simulink model "projection_test_4D"  (R2018b)
settings: Solver=VariableStepAuto  StartTime=0.0  StopTime=10.0  RelTol=1e-3
undefined symbols (not defined in the file): fswParams
libraries: simulink_extras x6, vrlib x2, L_inf_allocation_lib x1
settings Model: Creator=Taylor  LastModifiedBy=Taylor

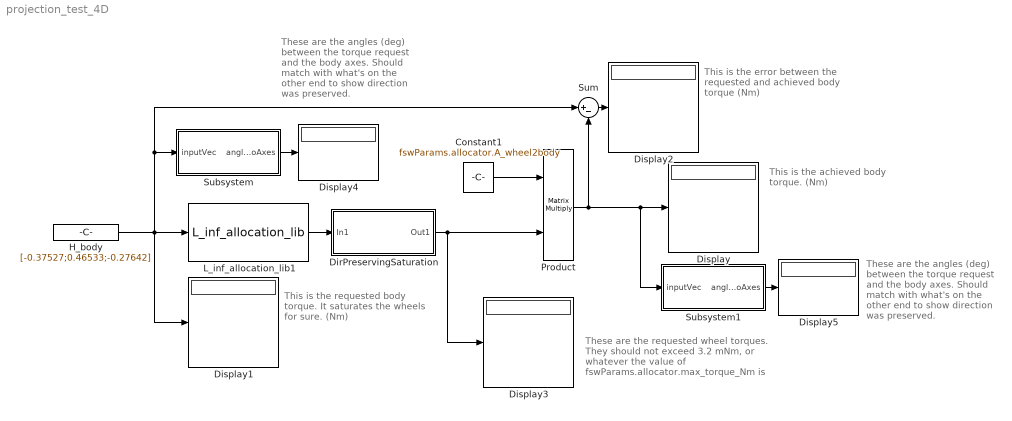
== system projection_test_4D ==
  note: This is the requested
      | body torque. It saturates
      | the wheels for sure. (Nm)
  note: This is the achieved
      | body torque. (Nm)
  note: These are the requested wheel
      | torques. They should not
      | exceed 3.2 mNm, or whatever
      | the value of
      | fswParams.allocator.max_torque_Nm
      | is
  note: These are the angles (deg)
      | between the torque
      | request and the body
      | axes. Should match
      | with what's on the
      | other end to show
      | direction was preserved.
  note: These are the angles (deg)
      | between the torque
      | request and the body
      | axes. Should match
      | with what's on the
      | other end to show
      | direction was preserved.
  note: This is the error between
      | the requested and achieved
      | body torque (Nm)
  Constant1 : Constant  Value=fswParams.allocator.A_wheel2body
  DirPreservingSaturation : Subsystem
  Display{,1..5} (6 alike) : Display
  H_body : Constant  Value=[-0.37527;0.46533;-0.27642]
  L_inf_allocation_lib1 : L_inf_allocation_lib/L_inf_allocation_lib  SystemSampleTime=-1
  Product : Product  Multiplication=Matrix(*)
  Subsystem : Subsystem
  Subsystem1 : Subsystem
  Sum : Sum  Inputs=|+-
  wires:
  Sum/1 -> Display2/1
  Constant1/1 -> Product/1
  H_body/1 -> Sum/1, Subsystem/1(inputVec), L_inf_allocation_lib1/1, Display1/1
  Product/1 -> Sum/2, Subsystem1/1(inputVec), Display/1
  L_inf_allocation_lib1/1 -> DirPreservingSaturation/1(In1)
  DirPreservingSaturation/1(Out1) -> Product/2, Display3/1
  Subsystem/1(anglesToAxes) -> Display4/1
  Subsystem1/1(anglesToAxes) -> Display5/1

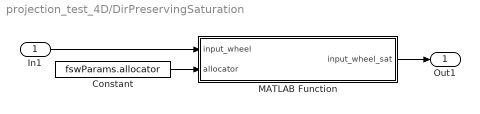
== system projection_test_4D/DirPreservingSaturation ==
  In1 : Inport
  Constant : Constant  Value=fswParams.allocator  OutDataTypeStr=Bus: RWA
  MATLAB Function : MATLAB Function  TreatAsAtomicUnit=on
  Out1 : Outport
  wires:
  MATLAB Function/1(input_wheel_sat) -> Out1/1
  In1/1 -> MATLAB Function/1(input_wheel)
  Constant/1 -> MATLAB Function/2(allocator)

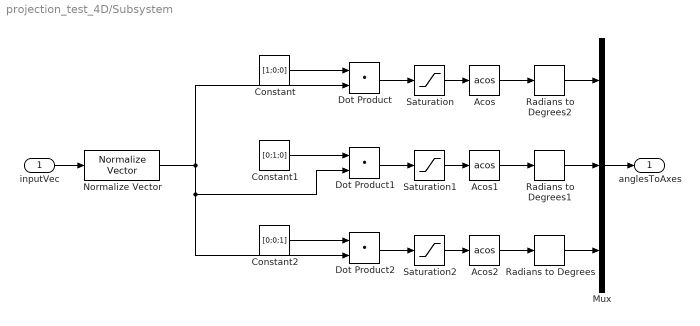
== system projection_test_4D/Subsystem ==
  inputVec : Inport
  Acos : Trigonometry  Operator=acos
  Acos1 : Trigonometry  Operator=acos
  Acos2 : Trigonometry  Operator=acos
  Constant : Constant  Value=[1;0;0]
  Constant1 : Constant  Value=[0;1;0]
  Constant2 : Constant  Value=[0;0;1]
  Dot Product : DotProduct  InputSameDT=on  OutDataTypeStr=Inherit: Inherit via internal rule
  Dot Product1 : DotProduct  InputSameDT=on  OutDataTypeStr=Inherit: Inherit via internal rule
  Dot Product2 : DotProduct  InputSameDT=on  OutDataTypeStr=Inherit: Inherit via internal rule
  Mux : Mux  Inputs=3
  Normalize Vector : vrlib/Utilities/Normalize Vector  maxzero=0
      settings: SourceProductName=Simulink 3D Animation  SourceProductBaseCode=VR
  Radians to Degrees : simulink_extras/Transformations/Radians to Degrees
  Radians to Degrees1 : simulink_extras/Transformations/Radians to Degrees
  Radians to Degrees2 : simulink_extras/Transformations/Radians to Degrees
  Saturation : Saturate  UpperLimit=1  LowerLimit=-1
  Saturation1 : Saturate  UpperLimit=1  LowerLimit=-1
  Saturation2 : Saturate  UpperLimit=1  LowerLimit=-1
  anglesToAxes : Outport
  wires:
  inputVec/1 -> Normalize Vector/1
  Normalize Vector/1 -> Dot Product2/2, Dot Product1/2, Dot Product/2
  Constant/1 -> Dot Product/1
  Constant1/1 -> Dot Product1/1
  Constant2/1 -> Dot Product2/1
  Dot Product/1 -> Saturation/1
  Dot Product1/1 -> Saturation1/1
  Dot Product2/1 -> Saturation2/1
  Saturation/1 -> Acos/1
  Saturation1/1 -> Acos1/1
  Saturation2/1 -> Acos2/1
  Acos2/1 -> Radians to Degrees/1
  Acos1/1 -> Radians to Degrees1/1
  Acos/1 -> Radians to Degrees2/1
  Radians to Degrees/1 -> Mux/3
  Radians to Degrees2/1 -> Mux/1
  Radians to Degrees1/1 -> Mux/2
  Mux/1 -> anglesToAxes/1

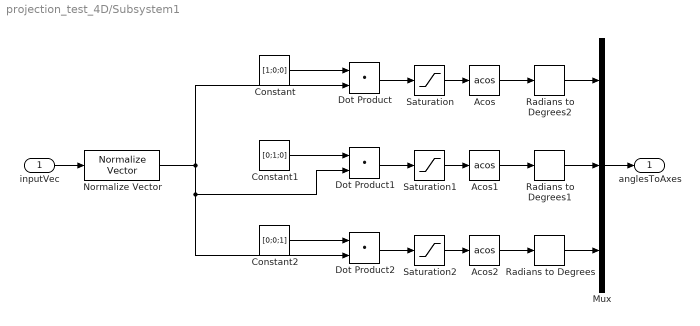
== system projection_test_4D/Subsystem1 ==
  inputVec : Inport
  Acos : Trigonometry  Operator=acos
  Acos1 : Trigonometry  Operator=acos
  Acos2 : Trigonometry  Operator=acos
  Constant : Constant  Value=[1;0;0]
  Constant1 : Constant  Value=[0;1;0]
  Constant2 : Constant  Value=[0;0;1]
  Dot Product : DotProduct  InputSameDT=on  OutDataTypeStr=Inherit: Inherit via internal rule
  Dot Product1 : DotProduct  InputSameDT=on  OutDataTypeStr=Inherit: Inherit via internal rule
  Dot Product2 : DotProduct  InputSameDT=on  OutDataTypeStr=Inherit: Inherit via internal rule
  Mux : Mux  Inputs=3
  Normalize Vector : vrlib/Utilities/Normalize Vector  maxzero=0
      settings: SourceProductName=Simulink 3D Animation  SourceProductBaseCode=VR
  Radians to Degrees : simulink_extras/Transformations/Radians to Degrees
  Radians to Degrees1 : simulink_extras/Transformations/Radians to Degrees
  Radians to Degrees2 : simulink_extras/Transformations/Radians to Degrees
  Saturation : Saturate  UpperLimit=1  LowerLimit=-1
  Saturation1 : Saturate  UpperLimit=1  LowerLimit=-1
  Saturation2 : Saturate  UpperLimit=1  LowerLimit=-1
  anglesToAxes : Outport
  wires:
  Mux/1 -> anglesToAxes/1
  Radians to Degrees1/1 -> Mux/2
  Radians to Degrees2/1 -> Mux/1
  Radians to Degrees/1 -> Mux/3
  Acos/1 -> Radians to Degrees2/1
  Acos1/1 -> Radians to Degrees1/1
  Acos2/1 -> Radians to Degrees/1
  Saturation2/1 -> Acos2/1
  Saturation1/1 -> Acos1/1
  Saturation/1 -> Acos/1
  Dot Product2/1 -> Saturation2/1
  Dot Product1/1 -> Saturation1/1
  Dot Product/1 -> Saturation/1
  Constant2/1 -> Dot Product2/1
  Constant1/1 -> Dot Product1/1
  Constant/1 -> Dot Product/1
  Normalize Vector/1 -> Dot Product/2, Dot Product1/2, Dot Product2/2
  inputVec/1 -> Normalize Vector/1

== matlab function projection_test_4D/DirPreservingSaturation/MATLAB Function ==
  data: input_wheel input; input_wheel_sat output; allocator input Bus: RWA
function input_wheel_sat = fcn(input_wheel,allocator)

In = eye(4);
A = [ In; -In ];
% b = allocator.max_torque_Nm .* ones(8,1);

temp = A*input_wheel-allocator.max_torque_Nm;
[val,id] = max(temp);

a = A(id,:);
b = allocator.max_torque_Nm;
c = dot(a,input_wheel);

if ( val > 0 )
    input_wheel_sat = (b/c) .* input_wheel;
else
    input_wheel_sat = input_wheel;
end

end
